simulink model "MagTest"  (R2021a)
settings: Solver=VariableStepAuto  StartTime=0.0  StopTime=5  RelTol=1e-3
libraries: simulink x3
settings Model: Creator=jmher  LastModifiedBy=jmher

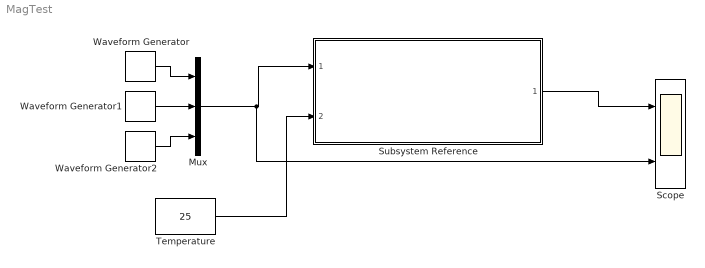
== system MagTest ==
  Mux : Mux  Inputs=3
  Scope : Scope  NumInputPorts=2
  Subsystem Reference : Subsystem  ReferencedSubsystem=Magnetometer
  Temperature : Constant  Value=25
  Waveform Generator : simulink/Sources/Waveform Generator  OutMin=[]  OutMax=[]  OutDataTypeStr=double  SelectedSignal=1  Signals=sin(30e-6, 1, 0)  BlockNames=MultiportSwitch_c694e09879574cb  SampleTime=0.1
  Waveform Generator1 : simulink/Sources/Waveform Generator  OutMin=[]  OutMax=[]  OutDataTypeStr=double  SelectedSignal=1  Signals=sin(30e-6, 1, 0)  BlockNames=MultiportSwitch_94a41e3cc8e14aa  SampleTime=0.1
  Waveform Generator2 : simulink/Sources/Waveform Generator  OutMin=[]  OutMax=[]  OutDataTypeStr=double  SelectedSignal=1  Signals=sin(30e-6, 1, 0)  BlockNames=MultiportSwitch_bc6494edc25d4f1  SampleTime=0.1
  wires:
  Subsystem Reference/1 -> Scope/1
  Waveform Generator2/1 -> Mux/3
  Waveform Generator1/1 -> Mux/2
  Waveform Generator/1 -> Mux/1
  Mux/1 -> Scope/2, Subsystem Reference/1
  Temperature/1 -> Subsystem Reference/2
